simulink model "real_MPC_schema"  (R2026a)
settings: Solver=ode4  FixedStep=pp.Ts_plant
values from neighbouring files (symbols this model uses):
  params =     [CEM_no_singularity_animation_data.mat]    (also in CEM_singularity_animation_data.mat; test_mpc_singularity_warning_sweep.m = baseParams)
settings Model: Creator=ryanj  LastModifiedBy=ryanj

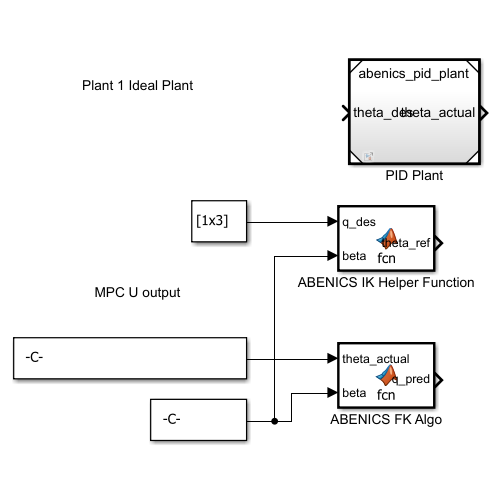
[thumbnail: Simulink's stored preview of the top-level diagram]
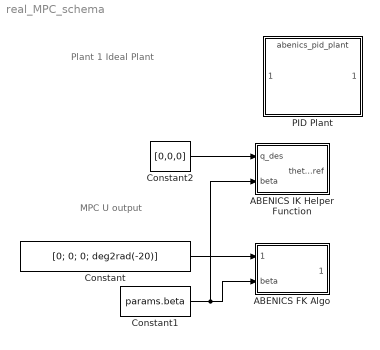
== system real_MPC_schema ==
  note: MPC U output
  note: Plant 1 Ideal Plant
  ABENICS FK Algo : MATLAB Function  TreatAsAtomicUnit=on
  ABENICS IK Helper Function : MATLAB Function  TreatAsAtomicUnit=on
  Constant : Constant  Value=[0; 0; 0; deg2rad(-20)]  SampleTime=params.Ts
  Constant1 : Constant  Value=params.beta  SampleTime=params.Ts
  Constant2 : Constant  Value=[0,0,0]  SampleTime=params.Ts
  PID Plant : ModelReference  ModelNameDialog=abenics_pid_plant  SimulationMode=Normal  ModelReferenceVersion=1.1
  wires:
  Constant2/1 -> ABENICS IK Helper Function/1(q_des)
  Constant/1 -> ABENICS FK Algo/1(theta_actual)
  Constant1/1 -> ABENICS IK Helper Function/2(beta), ABENICS FK Algo/2(beta)

== matlab function real_MPC_schema/ABENICS IK Helper Function ==
  data: q_des input; theta_ref output; beta input
function theta_ref = fcn(q_des, beta)
%#codegen

params.beta = beta;

theta_ref = abenicsIK(q_des, params);

end

== matlab function real_MPC_schema/ABENICS FK Algo ==
  data: theta_actual input size=[4,1]; q_pred output size=[3,1]; beta input
function q_pred = fcn(theta_actual, beta)
%#codegen

params.beta = beta;
q_pred = abenicsFK(theta_actual, params);

end
